simulink model "ASU_EC3_Supervisor"  (R2014a)
settings: Solver=ode45  StartTime=0.0  StopTime=10.0  RelTol=1e-3
libraries: simulink x14, dspsigattribs x1
settings Model: Creator=Megan  LastModifiedBy=Rashad

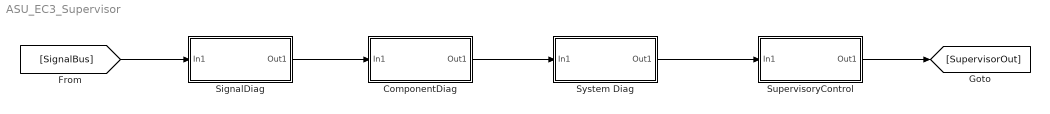
== system ASU_EC3_Supervisor ==
  ComponentDiag : Subsystem
  SignalDiag : Subsystem
  SupervisoryControl : Subsystem
  System Diag : Subsystem
  wires:
  [SignalBus] -> SignalDiag/1(In1)
  SignalDiag/1(Out1) -> ComponentDiag/1(In1)
  ComponentDiag/1(Out1) -> System Diag/1(In1)
  System Diag/1(Out1) -> SupervisoryControl/1(In1)
  SupervisoryControl/1(Out1) -> [SupervisorOut]

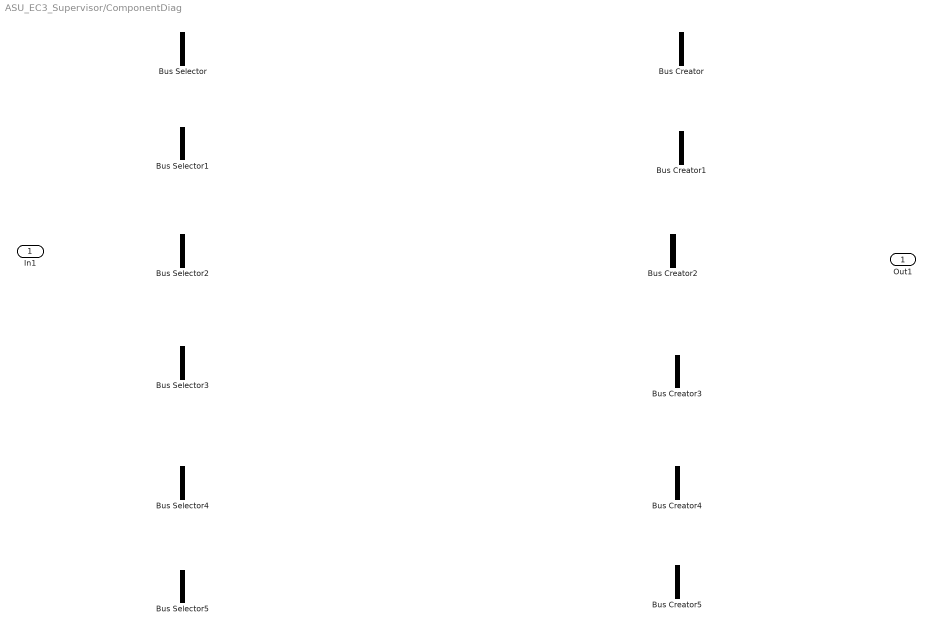
== system ASU_EC3_Supervisor/ComponentDiag ==
  In1 : Inport
  Bus Creator{,1..5} (6 alike) : BusCreator  Inputs=2
  Bus Selector{,1..5} (6 alike) : BusSelector  OutputSignals=signal1,signal2
  Out1 : Outport

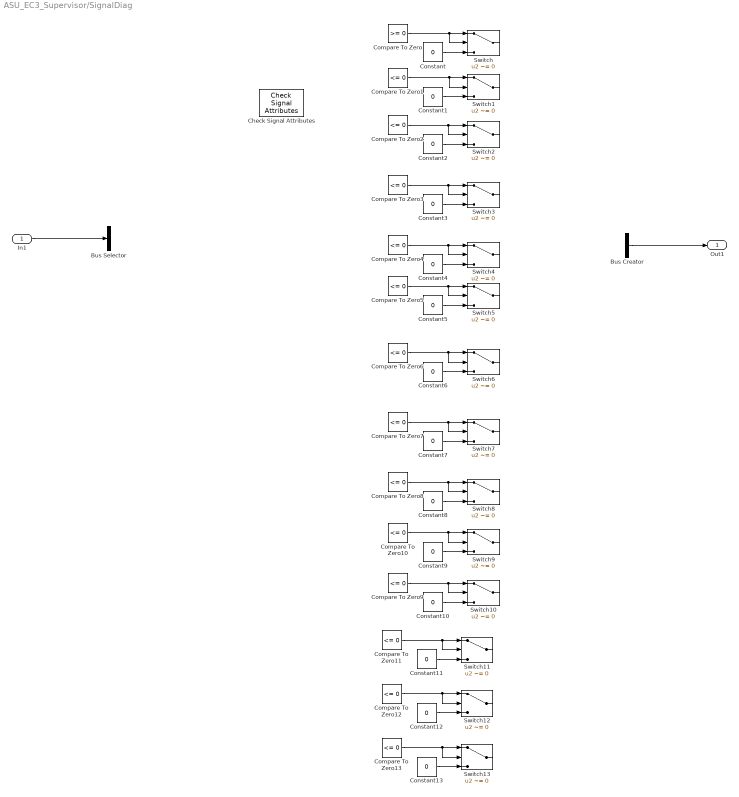
== system ASU_EC3_Supervisor/SignalDiag ==
  In1 : Inport
  Bus Creator : BusCreator  Inputs=2
  Bus Selector : BusSelector  OutputSignals=signal1,signal2
  Check Signal Attributes : dspsigattribs/Check Signal Attributes  SigAttribCheckMethod=Does not match attributes exactly  Complexity=Real  Frame=Ignore  DimsCheckMethod=Is...  Dimensions=Scalar (1-D or 2-D)  DatatypeCheckMethod=Ignore  DatatypeGeneral=Boolean  DtypeFloatSpecific=Any floating-point  DtypeFixedSpecific=Any fixed-point  DtypeIntSpecific=Any integer  SampleMode=Ignore
  Compare To Zero : simulink/Logic and Bit Operations/Compare To Zero  relop=>=  OutDataTypeStr=boolean
  Compare To Zero{1..13} (13 alike) : simulink/Logic and Bit Operations/Compare To Zero  relop=<=  OutDataTypeStr=boolean
  Constant{,1..13} (14 alike) : Constant  Value=0
  Switch{,1..13} (14 alike) : Switch  Criteria=u2 ~= 0
  Out1 : Outport
  wires:
  In1/1 -> Bus Selector/1
  Bus Creator/1 -> Out1/1
  Compare To Zero/1 -> Switch/2, Switch/1
  Constant/1 -> Switch/3
  Compare To Zero1/1 -> Switch1/1, Switch1/2
  Constant1/1 -> Switch1/3
  Compare To Zero2/1 -> Switch2/2, Switch2/1
  Constant2/1 -> Switch2/3
  Compare To Zero3/1 -> Switch3/1, Switch3/2
  Constant3/1 -> Switch3/3
  Compare To Zero4/1 -> Switch4/2, Switch4/1
  Constant4/1 -> Switch4/3
  Compare To Zero5/1 -> Switch5/1, Switch5/2
  Constant5/1 -> Switch5/3
  Compare To Zero6/1 -> Switch6/2, Switch6/1
  Constant6/1 -> Switch6/3
  Compare To Zero7/1 -> Switch7/1, Switch7/2
  Constant7/1 -> Switch7/3
  Compare To Zero8/1 -> Switch8/2, Switch8/1
  Constant8/1 -> Switch8/3
  Compare To Zero10/1 -> Switch9/1, Switch9/2
  Constant9/1 -> Switch9/3
  Compare To Zero9/1 -> Switch10/2, Switch10/1
  Constant10/1 -> Switch10/3
  Compare To Zero11/1 -> Switch11/1, Switch11/2
  Constant11/1 -> Switch11/3
  Compare To Zero12/1 -> Switch12/2, Switch12/1
  Constant12/1 -> Switch12/3
  Compare To Zero13/1 -> Switch13/1, Switch13/2
  Constant13/1 -> Switch13/3

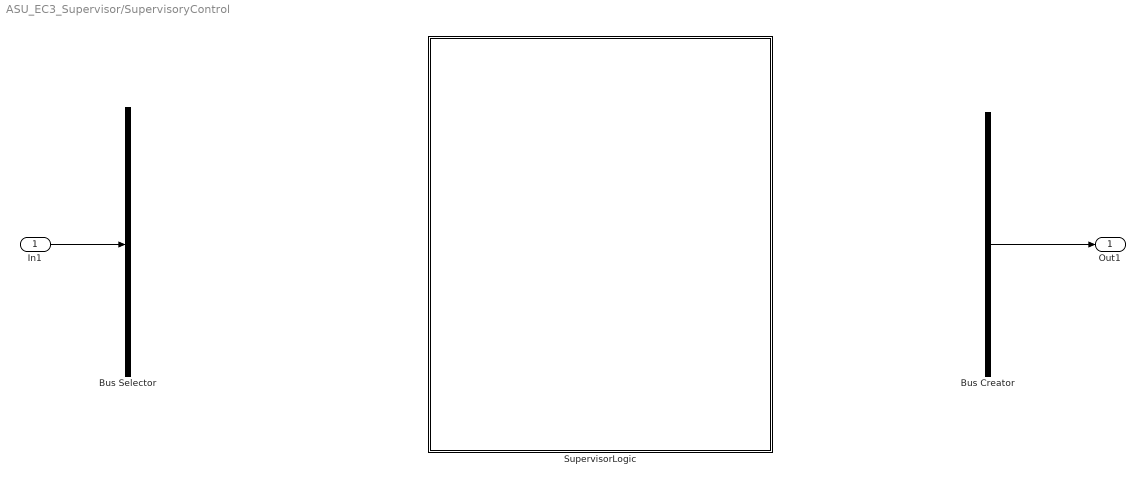
== system ASU_EC3_Supervisor/SupervisoryControl ==
  In1 : Inport
  Bus Creator : BusCreator  Inputs=2
  Bus Selector : BusSelector  OutputSignals=signal1,signal2
  SupervisorLogic : Stateflow chart  TreatAsAtomicUnit=on
  Out1 : Outport
  wires:
  In1/1 -> Bus Selector/1
  Bus Creator/1 -> Out1/1

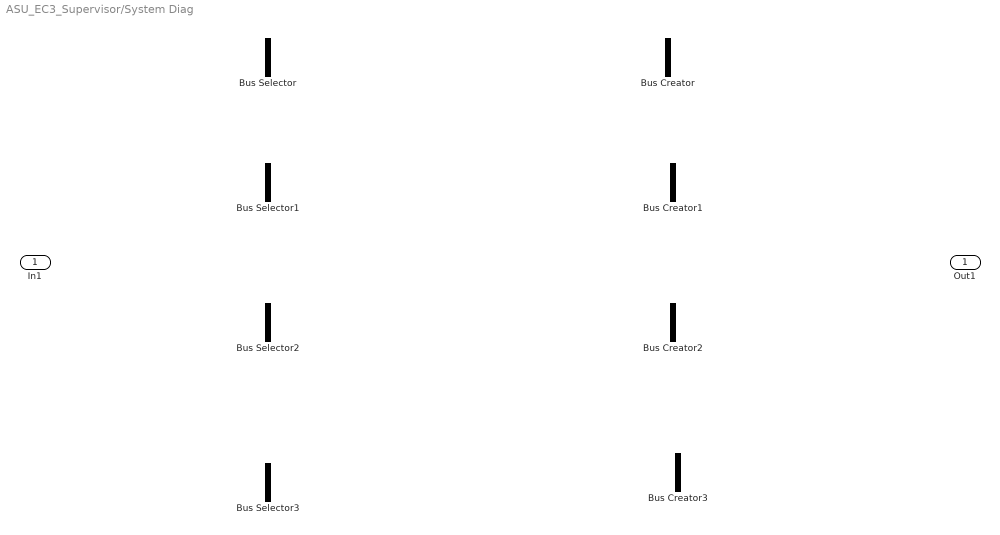
== system ASU_EC3_Supervisor/System Diag ==
  In1 : Inport
  Bus Creator{,1..3} (4 alike) : BusCreator  Inputs=2
  Bus Selector{,1..3} (4 alike) : BusSelector  OutputSignals=signal1,signal2
  Out1 : Outport

== stateflow chart ASU_EC3_Supervisor/SupervisoryControl/SupervisorLogic ==
  state Drivelogic [parallel]
    settings: executionOrder=1
    state VehicleOfforAcc
    state Shutdown
    state Startup
    state VehicleReady
      state PerformanceDrive
      state NormalDrive
        state EVOnly
          state Accel
          state Brake_Idle
          Drivelogic.VehicleReady.NormalDrive.EVOnly.Accel -> Drivelogic.VehicleReady.NormalDrive.EVOnly.Brake_Idle
          Drivelogic.VehicleReady.NormalDrive.EVOnly.Brake_Idle -> Drivelogic.VehicleReady.NormalDrive.EVOnly.Accel
        state ICEOnly
          state Accel
          state Brake_Idle
        state HEV
          state CD
          state CS
          state Brake_Idle
        EVOnly -> ICEOnly [order 2]
        ICEOnly -> EVOnly [order 2]
        EVOnly -> HEV [order 1]
        HEV -> EVOnly [order 1]
        ICEOnly -> HEV [order 1]
        HEV -> ICEOnly [order 2]
      NormalDrive -> PerformanceDrive
      PerformanceDrive -> NormalDrive
    VehicleOfforAcc -> Startup
    Startup -> VehicleOfforAcc [order 2]
    Shutdown -> VehicleOfforAcc
    VehicleReady -> Shutdown
    Startup -> VehicleReady [order 1]
  state EngineTime [parallel]
    settings: executionOrder=2
  state EngineON [parallel]
    settings: executionOrder=3
  state Clutch [parallel]
    settings: executionOrder=4
